simulink model "untitled"  (R2023a)
settings: Solver=VariableStepAuto  StartTime=0.0  StopTime=1  RelTol=1e-3
settings Model: Creator=satalofs  LastModifiedBy=satalofs

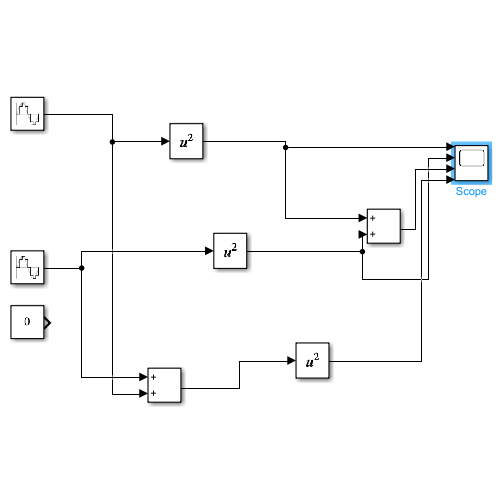
[thumbnail: Simulink's stored preview of the top-level diagram]
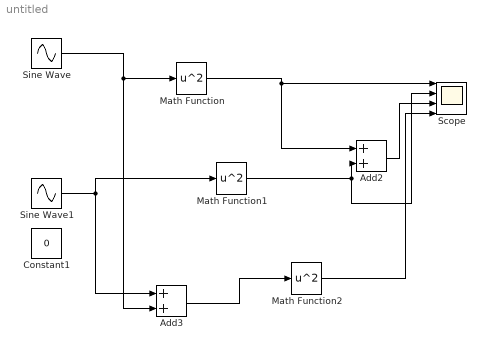
== system untitled ==
  Add2 : Sum
  Add3 : Sum
  Constant1 : Constant  Value=0
  Math Function : Math  Operator=square
  Math Function1 : Math  Operator=square
  Math Function2 : Math  Operator=square
  Scope : Scope  NumInputPorts=4
  Sine Wave : Sin  Frequency=2*pi*20  SampleTime=1/2000
  Sine Wave1 : Sin  Frequency=2*pi*30  SampleTime=1/2000
  wires:
  Sine Wave/1 -> Math Function/1, Add3/2
  Sine Wave1/1 -> Add3/1, Math Function1/1
  Math Function1/1 -> Scope/2, Add2/2
  Add2/1 -> Scope/3
  Add3/1 -> Math Function2/1
  Math Function2/1 -> Scope/4
  Math Function/1 -> Add2/1, Scope/1
